simulink model "UAVtree21"  (R2019b)
settings: Solver=FixedStepAuto  StartTime=0.0  StopTime=50  RelTol=1e-3
undefined symbols (not defined in the file or in its folder): DiscIntNeverNeededParam
libraries: simulink x5, vrlib x4, robotcorelib x1
settings Model: Creator=Tesla  LastModifiedBy=Tesla
settings OptimizationCC: OptimizeBlockIOStorage=off  BufferReuse=off  GlobalBufferReuse=off  ExpressionFolding=off  LocalBlockOutputs=off  OptimizeDataStoreBuffers=off  BusAssignmentInplaceUpdate=off
settings DebuggingCC: SFUnexpectedBacktrackingDiag=warning  SFNoUnconditionalDefaultTransitionDiag=warning  UnderSpecifiedDimensionMsg=warning
settings RTWCC: GenerateReport=on  BuildConfiguration=Debug  LaunchReport=on  TargetLang=C++
settings CodeAppCC: ForceParamTrailComments=on  MATLABSourceComments=on  EnableCustomComments=on
settings GRTTargetCC: TargetLangStandard=C++03 (ISO)  CombineSignalStateStructs=on  MultiInstanceERTCode=on  CodeInterfacePackaging=C++ class  SupportVariableSizeSignals=on  MultiInstanceErrorCode=Warning

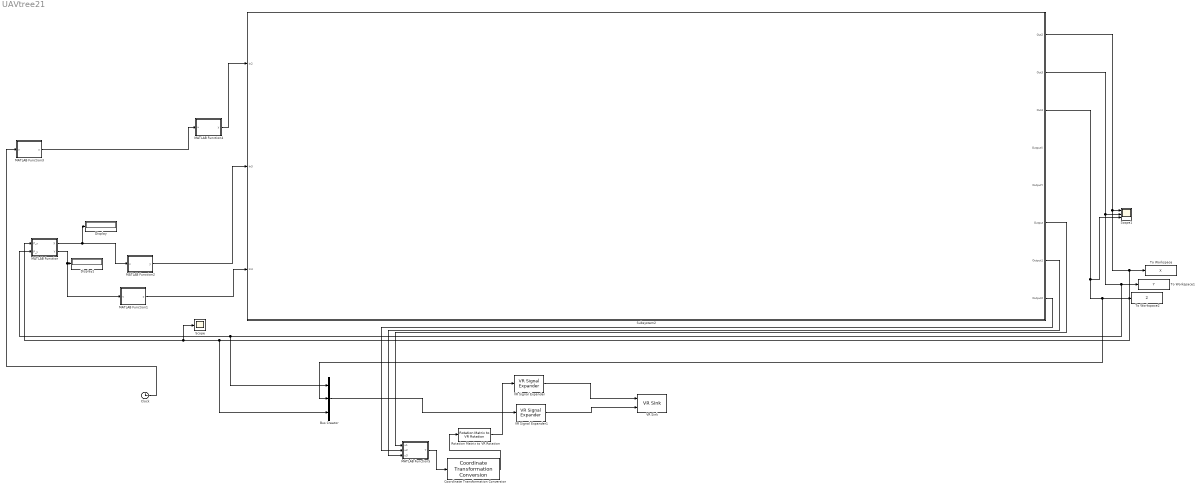
== system UAVtree21 ==
  Bus Creator : BusCreator  Inputs=3
  Clock : Clock
  Coordinate Transformation Conversion : robotcorelib/Coordinate Transformation Conversion  InputRepresentation=Euler Angles  InputEulerSequence=XYZ  ShowTrVecInputPort=on  OutputRepresentation=Rotation Matrix  OutputEulerSequence=ZYX  ShowTrVecOutputPort=on  SimulateUsing=Interpreted execution
      settings: SourceProductBaseCode=RO
  Display : Display
  Display1 : Display
  MATLAB Function : MATLAB Function  TreatAsAtomicUnit=on
  MATLAB Function1 : MATLAB Function  TreatAsAtomicUnit=on
  MATLAB Function2 : MATLAB Function  TreatAsAtomicUnit=on
  MATLAB Function3 : MATLAB Function  TreatAsAtomicUnit=on
  MATLAB Function4 : MATLAB Function  TreatAsAtomicUnit=on
  MATLAB Function5 : MATLAB Function  TreatAsAtomicUnit=on
  Rotation Matrix to VR Rotation : vrlib/Utilities/Rotation Matrix to VR Rotation  maxzero=1e-5
      settings: SourceProductName=Simulink  SourceProductBaseCode=SL
  Scope : Scope
  Scope1 : Scope  NumInputPorts=3
  Subsystem2 : Subsystem
  To Workspace : ToWorkspace  VariableName=X  SampleTime=-1
  To Workspace1 : ToWorkspace  VariableName=Y  SampleTime=-1
  To Workspace2 : ToWorkspace  VariableName=Z  SampleTime=-1
  VR Signal Expander : vrlib/VR Signal Expander  outwidth=4  outidx=[1 2 3 4]
      settings: SourceProductName=Simulink
  VR Signal Expander1 : vrlib/VR Signal Expander  outwidth=3  outidx=[1 2 3]
      settings: SourceProductName=Simulink
  VR Sink : vrlib/VR Sink  InstantiateOnLoad=on  SampleTime=0.005  ViewEnable=on  RemoteChange=off  RemoteView=off  FieldsWritten=vehicle.rotation.4.1.1.double#vehicle.translation.3.1.1.double  WorldFileName=advance.wrl  AutoView=on  VideoDimensions=[]  AllowVariableSize=off
      settings: SourceProductName=Simulink
  wires:
  Subsystem2/2(Out3) -> Scope1/2, Bus Creator/1, MATLAB Function/2(P_y), To Workspace1/1
  Subsystem2/3(Out4) -> Bus Creator/2, To Workspace2/1, Scope1/3
  MATLAB Function/2(Y) -> MATLAB Function1/1(u), Display1/1
  MATLAB Function/1(X) -> MATLAB Function2/1(u), Display/1
  MATLAB Function1/1(y) -> Subsystem2/3(In4)
  MATLAB Function2/1(y) -> Subsystem2/2(In3)
  Subsystem2/1(Out2) -> Scope1/1, Bus Creator/3, MATLAB Function/1(P_x), Scope/1, To Workspace/1
  Clock/1 -> MATLAB Function3/1(u)
  MATLAB Function3/1(y) -> MATLAB Function4/1(u)
  MATLAB Function4/1(y) -> Subsystem2/1(In2)
  Bus Creator/1 -> VR Signal Expander1/1
  Subsystem2/6(Output) -> MATLAB Function5/1(u1)
  Subsystem2/7(Output1) -> MATLAB Function5/3(u3)
  Subsystem2/8(Output2) -> MATLAB Function5/2(u2)
  MATLAB Function5/1(Y) -> Coordinate Transformation Conversion/1
  Rotation Matrix to VR Rotation/1 -> VR Signal Expander/1
  Coordinate Transformation Conversion/1 -> Rotation Matrix to VR Rotation/1
  VR Signal Expander/1 -> VR Sink/1
  VR Signal Expander1/1 -> VR Sink/2

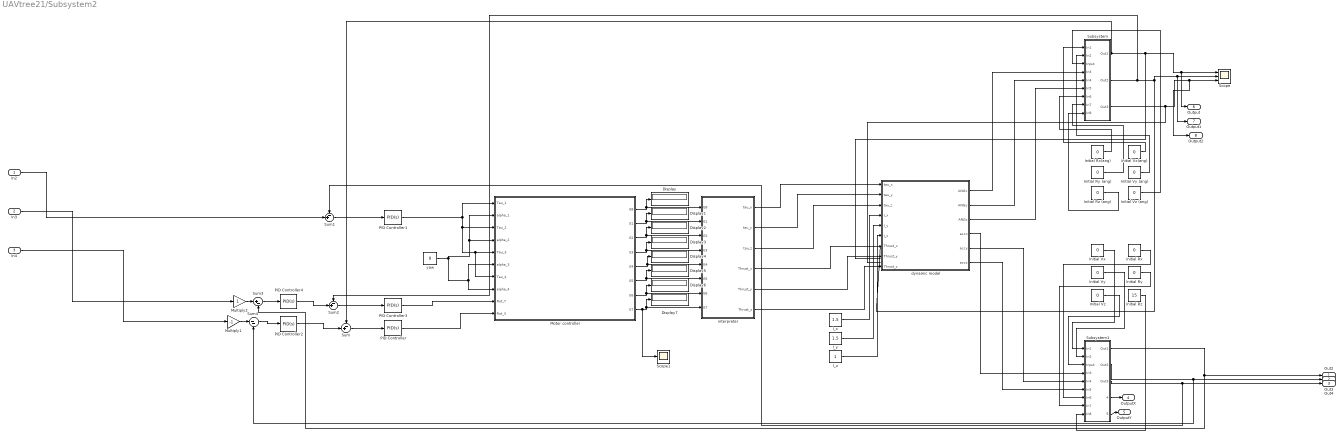
== system UAVtree21/Subsystem2 ==
  In2 : Inport
  In3 : Inport  Port=2
  In4 : Inport  Port=3
  Display{,1..7} (8 alike) : Display
  I_x : Constant  Value=1.5
  I_y : Constant  Value=1.5
  I_z : Constant
  Initial Rx : Constant  Value=0
  Initial Rx(ang) : Constant  Value=0
  Initial Ry : Constant  Value=0
  Initial Ry (ang) : Constant  Value=0
  Initial Rz : Constant  Value=15
  Initial Rz (ang) : Constant  Value=0
  Initial Vx : Constant  Value=0
  Initial Vx(ang) : Constant  Value=0
  "Initial Vy " : Constant  Value=0
  Initial Vy (ang) : Constant  Value=0
  Initial Vz : Constant  Value=0
  Initial Vz (ang) : Constant  Value=0
  Motor controller : Subsystem
  Multiply1 : Gain  Gain=-1
  Multiply2 : Gain
  PID Controller : simulink/Continuous/PID Controller  Controller=PID  Form=Parallel  TimeDomain=Continuous-time  SampleTime=-1  IntegratorMethod=Forward Euler  FilterMethod=Forward Euler  ControllerParametersSource=internal  P=-19  I=-5  D=-8  UseFilter=on  N=25  TunerSelectOption=Transfer Function Based (PID Tuner App)  InitialConditionSource=internal  InitialConditionForIntegrator=0  InitialConditionForFilter=0  DifferentiatorICPrevScaledInput=0  ExternalReset=none  TrackingMode=off  Kt=1  LimitOutput=on  UpperSaturationLimit=2  LowerSaturationLimit=-2  LinearizeAsGain=on  AntiWindupMode=clamping  Kb=1  POutMin=[]  POutMax=[]  IOutMin=[]  IOutMax=[]  DOutMin=[]  DOutMax=[]  NOutMin=[]  NOutMax=[]  SumOutMin=[]  SumOutMax=[]  SaturationOutMin=[]  SaturationOutMax=[]  PParamMin=[]  PParamMax=[]  IParamMin=[]  IParamMax=[]  DParamMin=[]  DParamMax=[]  NParamMin=[]  NParamMax=[]  KbParamMin=[]  KbParamMax=[]  KtParamMin=[]  KtParamMax=[]  KbOutMin=[]  KbOutMax=[]  KtOutMin=[]  KtOutMax=[]  IntegratorOutMin=[]  IntegratorOutMax=[]  FilterOutMin=[]  FilterOutMax=[]  SumI1OutMin=[]  SumI1OutMax=[]  SumI2OutMin=[]  SumI2OutMax=[]  SumI3OutMin=[]  SumI3OutMax=[]  SumI4OutMin=[]  SumI4OutMax=[]  SumDOutMin=[]  SumDOutMax=[]  DifferentiatorOutMin=[]  DifferentiatorOutMax=[]  FilterDiffOutCoefMin=[]  FilterDiffOutCoefMax=[]  ReciprocalOutMin=[]  ReciprocalOutMax=[]  SumDenOutMin=[]  SumDenOutMax=[]  SumNumOutMin=[]  SumNumOutMax=[]  DivideOutMin=[]  DivideOutMax=[]  IntegratorContinuousStateAttributes=''  IntegratorStateMustResolveToSignalObject=off  IntegratorRTWStateStorageClass=Auto  FilterContinuousStateAttributes=''  FilterStateMustResolveToSignalObject=off  FilterRTWStateStorageClass=Auto  ParallelPVariant=InternalParameters  IdealPVariant=Disabled  IVariant=InternalParameters  DVariant=InternalParameters  IntegratorVariant=Continuous  SatVariant=Enabled  AWVariant=ContClampingParallel  PCopyVariant=Disabled  TRVariant=Disabled  FdbkBlocksVariant=Forward  IdealPFdbkVariant=Disabled  SatFdbkVariant=Disabled  DerivativeFilterVariant=ContFilter  NVariant=InternalParameters  NCopyVariant=Disabled  FilterICVariant=InternalICsFilter  IntegratorICVariant=InternalICs  ExternalResetVariant=Disabled  TRSumVariant=Passthrough  SumFdbkVariant=Disabled  SumVariant=Sum_PID
  PID Controller1 : simulink/Continuous/PID Controller  Controller=PID  Form=Parallel  TimeDomain=Continuous-time  SampleTime=-1  IntegratorMethod=Forward Euler  FilterMethod=Forward Euler  ControllerParametersSource=internal  P=65  I=50  D=40  UseFilter=on  N=25  TunerSelectOption=Frequency Response Based  InitialConditionSource=internal  InitialConditionForIntegrator=0  InitialConditionForFilter=0  DifferentiatorICPrevScaledInput=0  ExternalReset=none  TrackingMode=off  Kt=1  LimitOutput=on  UpperSaturationLimit=12  LowerSaturationLimit=0  LinearizeAsGain=off  AntiWindupMode=clamping  Kb=1  POutMin=[]  POutMax=[]  IOutMin=[]  IOutMax=[]  DOutMin=[]  DOutMax=[]  NOutMin=[]  NOutMax=[]  SumOutMin=[]  SumOutMax=[]  SaturationOutMin=[]  SaturationOutMax=[]  PParamMin=[]  PParamMax=[]  IParamMin=[]  IParamMax=[]  DParamMin=[]  DParamMax=[]  NParamMin=[]  NParamMax=[]  KbParamMin=[]  KbParamMax=[]  KtParamMin=[]  KtParamMax=[]  KbOutMin=[]  KbOutMax=[]  KtOutMin=[]  KtOutMax=[]  IntegratorOutMin=[]  IntegratorOutMax=[]  FilterOutMin=[]  FilterOutMax=[]  SumI1OutMin=[]  SumI1OutMax=[]  SumI2OutMin=[]  SumI2OutMax=[]  SumI3OutMin=[]  SumI3OutMax=[]  SumI4OutMin=[]  SumI4OutMax=[]  SumDOutMin=[]  SumDOutMax=[]  DifferentiatorOutMin=[]  DifferentiatorOutMax=[]  FilterDiffOutCoefMin=[]  FilterDiffOutCoefMax=[]  ReciprocalOutMin=[]  ReciprocalOutMax=[]  SumDenOutMin=[]  SumDenOutMax=[]  SumNumOutMin=[]  SumNumOutMax=[]  DivideOutMin=[]  DivideOutMax=[]  IntegratorContinuousStateAttributes=''  IntegratorStateMustResolveToSignalObject=off  IntegratorRTWStateStorageClass=Auto  FilterContinuousStateAttributes=''  FilterStateMustResolveToSignalObject=off  FilterRTWStateStorageClass=Auto  ParallelPVariant=InternalParameters  IdealPVariant=Disabled  IVariant=InternalParameters  DVariant=InternalParameters  IntegratorVariant=Continuous  SatVariant=Enabled  AWVariant=ContClampingParallel  PCopyVariant=Disabled  TRVariant=Disabled  FdbkBlocksVariant=Forward  IdealPFdbkVariant=Disabled  SatFdbkVariant=Disabled  DerivativeFilterVariant=ContFilter  NVariant=InternalParameters  NCopyVariant=Disabled  FilterICVariant=InternalICsFilter  IntegratorICVariant=InternalICs  ExternalResetVariant=Disabled  TRSumVariant=Passthrough  SumFdbkVariant=Disabled  SumVariant=Sum_PID
  PID Controller2 : simulink/Continuous/PID Controller  Controller=PID  Form=Parallel  TimeDomain=Continuous-time  SampleTime=-1  IntegratorMethod=Forward Euler  FilterMethod=Forward Euler  ControllerParametersSource=internal  P=-0.3  I=-0.01  D=-0.025  UseFilter=on  N=100  TunerSelectOption=Transfer Function Based (PID Tuner App)  InitialConditionSource=internal  InitialConditionForIntegrator=0  InitialConditionForFilter=0  DifferentiatorICPrevScaledInput=0  ExternalReset=none  TrackingMode=off  Kt=1  LimitOutput=on  UpperSaturationLimit=1  LowerSaturationLimit=-1  LinearizeAsGain=on  AntiWindupMode=clamping  Kb=1  POutMin=[]  POutMax=[]  IOutMin=[]  IOutMax=[]  DOutMin=[]  DOutMax=[]  NOutMin=[]  NOutMax=[]  SumOutMin=[]  SumOutMax=[]  SaturationOutMin=[]  SaturationOutMax=[]  PParamMin=[]  PParamMax=[]  IParamMin=[]  IParamMax=[]  DParamMin=[]  DParamMax=[]  NParamMin=[]  NParamMax=[]  KbParamMin=[]  KbParamMax=[]  KtParamMin=[]  KtParamMax=[]  KbOutMin=[]  KbOutMax=[]  KtOutMin=[]  KtOutMax=[]  IntegratorOutMin=[]  IntegratorOutMax=[]  FilterOutMin=[]  FilterOutMax=[]  SumI1OutMin=[]  SumI1OutMax=[]  SumI2OutMin=[]  SumI2OutMax=[]  SumI3OutMin=[]  SumI3OutMax=[]  SumI4OutMin=[]  SumI4OutMax=[]  SumDOutMin=[]  SumDOutMax=[]  DifferentiatorOutMin=[]  DifferentiatorOutMax=[]  FilterDiffOutCoefMin=[]  FilterDiffOutCoefMax=[]  ReciprocalOutMin=[]  ReciprocalOutMax=[]  SumDenOutMin=[]  SumDenOutMax=[]  SumNumOutMin=[]  SumNumOutMax=[]  DivideOutMin=[]  DivideOutMax=[]  IntegratorContinuousStateAttributes=''  IntegratorStateMustResolveToSignalObject=off  IntegratorRTWStateStorageClass=Auto  FilterContinuousStateAttributes=''  FilterStateMustResolveToSignalObject=off  FilterRTWStateStorageClass=Auto  ParallelPVariant=InternalParameters  IdealPVariant=Disabled  IVariant=InternalParameters  DVariant=InternalParameters  IntegratorVariant=Continuous  SatVariant=Enabled  AWVariant=ContClampingParallel  PCopyVariant=Disabled  TRVariant=Disabled  FdbkBlocksVariant=Forward  IdealPFdbkVariant=Disabled  SatFdbkVariant=Disabled  DerivativeFilterVariant=ContFilter  NVariant=InternalParameters  NCopyVariant=Disabled  FilterICVariant=InternalICsFilter  IntegratorICVariant=InternalICs  ExternalResetVariant=Disabled  TRSumVariant=Passthrough  SumFdbkVariant=Disabled  SumVariant=Sum_PID
  PID Controller3 : simulink/Continuous/PID Controller  Controller=PID  Form=Parallel  TimeDomain=Continuous-time  SampleTime=-1  IntegratorMethod=Forward Euler  FilterMethod=Forward Euler  ControllerParametersSource=internal  P=19  I=5  D=8  UseFilter=on  N=25  TunerSelectOption=Transfer Function Based (PID Tuner App)  InitialConditionSource=internal  InitialConditionForIntegrator=0  InitialConditionForFilter=0  DifferentiatorICPrevScaledInput=0  ExternalReset=none  TrackingMode=off  Kt=1  LimitOutput=on  UpperSaturationLimit=2  LowerSaturationLimit=-2  LinearizeAsGain=on  AntiWindupMode=clamping  Kb=1  POutMin=[]  POutMax=[]  IOutMin=[]  IOutMax=[]  DOutMin=[]  DOutMax=[]  NOutMin=[]  NOutMax=[]  SumOutMin=[]  SumOutMax=[]  SaturationOutMin=[]  SaturationOutMax=[]  PParamMin=[]  PParamMax=[]  IParamMin=[]  IParamMax=[]  DParamMin=[]  DParamMax=[]  NParamMin=[]  NParamMax=[]  KbParamMin=[]  KbParamMax=[]  KtParamMin=[]  KtParamMax=[]  KbOutMin=[]  KbOutMax=[]  KtOutMin=[]  KtOutMax=[]  IntegratorOutMin=[]  IntegratorOutMax=[]  FilterOutMin=[]  FilterOutMax=[]  SumI1OutMin=[]  SumI1OutMax=[]  SumI2OutMin=[]  SumI2OutMax=[]  SumI3OutMin=[]  SumI3OutMax=[]  SumI4OutMin=[]  SumI4OutMax=[]  SumDOutMin=[]  SumDOutMax=[]  DifferentiatorOutMin=[]  DifferentiatorOutMax=[]  FilterDiffOutCoefMin=[]  FilterDiffOutCoefMax=[]  ReciprocalOutMin=[]  ReciprocalOutMax=[]  SumDenOutMin=[]  SumDenOutMax=[]  SumNumOutMin=[]  SumNumOutMax=[]  DivideOutMin=[]  DivideOutMax=[]  IntegratorContinuousStateAttributes=''  IntegratorStateMustResolveToSignalObject=off  IntegratorRTWStateStorageClass=Auto  FilterContinuousStateAttributes=''  FilterStateMustResolveToSignalObject=off  FilterRTWStateStorageClass=Auto  ParallelPVariant=InternalParameters  IdealPVariant=Disabled  IVariant=InternalParameters  DVariant=InternalParameters  IntegratorVariant=Continuous  SatVariant=Enabled  AWVariant=ContClampingParallel  PCopyVariant=Disabled  TRVariant=Disabled  FdbkBlocksVariant=Forward  IdealPFdbkVariant=Disabled  SatFdbkVariant=Disabled  DerivativeFilterVariant=ContFilter  NVariant=InternalParameters  NCopyVariant=Disabled  FilterICVariant=InternalICsFilter  IntegratorICVariant=InternalICs  ExternalResetVariant=Disabled  TRSumVariant=Passthrough  SumFdbkVariant=Disabled  SumVariant=Sum_PID
  PID Controller4 : simulink/Continuous/PID Controller  Controller=PID  Form=Parallel  TimeDomain=Continuous-time  SampleTime=-1  IntegratorMethod=Forward Euler  FilterMethod=Forward Euler  ControllerParametersSource=internal  P=-0.3  I=-0.01  D=-0.025  UseFilter=on  N=150  TunerSelectOption=Transfer Function Based (PID Tuner App)  InitialConditionSource=internal  InitialConditionForIntegrator=0  InitialConditionForFilter=0  DifferentiatorICPrevScaledInput=0  ExternalReset=none  TrackingMode=off  Kt=1  LimitOutput=on  UpperSaturationLimit=1  LowerSaturationLimit=-1  LinearizeAsGain=off  AntiWindupMode=clamping  Kb=1  POutMin=[]  POutMax=[]  IOutMin=[]  IOutMax=[]  DOutMin=[]  DOutMax=[]  NOutMin=[]  NOutMax=[]  SumOutMin=[]  SumOutMax=[]  SaturationOutMin=[]  SaturationOutMax=[]  PParamMin=[]  PParamMax=[]  IParamMin=[]  IParamMax=[]  DParamMin=[]  DParamMax=[]  NParamMin=[]  NParamMax=[]  KbParamMin=[]  KbParamMax=[]  KtParamMin=[]  KtParamMax=[]  KbOutMin=[]  KbOutMax=[]  KtOutMin=[]  KtOutMax=[]  IntegratorOutMin=[]  IntegratorOutMax=[]  FilterOutMin=[]  FilterOutMax=[]  SumI1OutMin=[]  SumI1OutMax=[]  SumI2OutMin=[]  SumI2OutMax=[]  SumI3OutMin=[]  SumI3OutMax=[]  SumI4OutMin=[]  SumI4OutMax=[]  SumDOutMin=[]  SumDOutMax=[]  DifferentiatorOutMin=[]  DifferentiatorOutMax=[]  FilterDiffOutCoefMin=[]  FilterDiffOutCoefMax=[]  ReciprocalOutMin=[]  ReciprocalOutMax=[]  SumDenOutMin=[]  SumDenOutMax=[]  SumNumOutMin=[]  SumNumOutMax=[]  DivideOutMin=[]  DivideOutMax=[]  IntegratorContinuousStateAttributes=''  IntegratorStateMustResolveToSignalObject=off  IntegratorRTWStateStorageClass=Auto  FilterContinuousStateAttributes=''  FilterStateMustResolveToSignalObject=off  FilterRTWStateStorageClass=Auto  ParallelPVariant=InternalParameters  IdealPVariant=Disabled  IVariant=InternalParameters  DVariant=InternalParameters  IntegratorVariant=Continuous  SatVariant=Enabled  AWVariant=ContClampingParallel  PCopyVariant=Disabled  TRVariant=Disabled  FdbkBlocksVariant=Forward  IdealPFdbkVariant=Disabled  SatFdbkVariant=Disabled  DerivativeFilterVariant=ContFilter  NVariant=InternalParameters  NCopyVariant=Disabled  FilterICVariant=InternalICsFilter  IntegratorICVariant=InternalICs  ExternalResetVariant=Disabled  TRSumVariant=Passthrough  SumFdbkVariant=Disabled  SumVariant=Sum_PID
  Scope : Scope  NumInputPorts=3
  Scope1 : Scope
  Subsystem : Subsystem
  Subsystem1 : Subsystem
  Sum : Sum  Inputs=-+|
  Sum1 : Sum  Inputs=-+|
  Sum2 : Sum  Inputs=-+|
  Sum3 : Sum  Inputs=|+-
  Sum4 : Sum  Inputs=|--
  dynamic model : MATLAB Function  TreatAsAtomicUnit=on
  interpreter : MATLAB Function  TreatAsAtomicUnit=on
  yaw : Constant  Value=0
  Out2 : Outport
  Out3 : Outport  Port=2
  Out4 : Outport  Port=3
  OutputX : Outport  Port=4
  OutputY : Outport  Port=5
  Output : Outport  Port=6
  Output1 : Outport  Port=7
  Output2 : Outport  Port=8
  wires:
  In3/1 -> Multiply2/1
  "Initial Vy "/1 -> Subsystem1/2(In2)
  Motor controller/2(E1) -> Display1/1, interpreter/2(E1)
  PID Controller1/1 -> Motor controller/5(Tau_3), Motor controller/7(Tau_4), Motor controller/3(Tau_2), Motor controller/1("Tau_1 ")
  Initial Rx(ang)/1 -> Subsystem/7(In6)
  Sum/1 -> PID Controller/1
  Subsystem1/2(Out2) -> Out3/1, Sum4/2
  Motor controller/5(E4) -> Display4/1, interpreter/5(E4)
  Subsystem1/1(Out1) -> Out2/1, Sum3/2
  Initial Vz/1 -> Subsystem1/3(Input)
  PID Controller2/1 -> Sum/2
  PID Controller/1 -> Motor controller/10(Rot_X)
  Motor controller/6(E5) -> Display5/1, interpreter/6(E5)
  Initial Vx(ang)/1 -> Subsystem/1(In1)
  dynamic model/2(ANGy) -> Subsystem/5(In4)
  dynamic model/4(accx) -> Subsystem1/4(In3)
  Subsystem/2(Out2) -> Sum2/1, Scope/2, Output1/1
  dynamic model/6(accz) -> Subsystem1/6(In5)
  Subsystem1/3(Out3) -> Out4/1, Sum1/1
  I_z/1 -> dynamic model/6(I_z)
  PID Controller4/1 -> Sum2/2
  Sum3/1 -> PID Controller4/1
  Initial Ry/1 -> Subsystem1/8(In7)
  Initial Vz (ang)/1 -> Subsystem/3(Input)
  Motor controller/1("E8 ") -> Display/1, interpreter/1(E8)
  Sum1/1 -> PID Controller1/1
  interpreter/1(tau_x) -> dynamic model/1(tau_x)
  Initial Vx/1 -> Subsystem1/1(In1)
  In4/1 -> Multiply1/1
  Initial Ry (ang)/1 -> Subsystem/8(In7)
  Subsystem/1(Out1) -> Scope/1, Output/1, Sum/1
  I_y/1 -> dynamic model/5(I_y)
  Sum2/1 -> PID Controller3/1
  Motor controller/7(E6) -> Display6/1, interpreter/7(E6)
  dynamic model/3(ANGz) -> Subsystem/6(In5)
  Sum4/1 -> PID Controller2/1
  Motor controller/8(E7) -> Scope1/1, Display7/1, interpreter/8(E7)
  Initial Rx/1 -> Subsystem1/7(In6)
  I_x/1 -> dynamic model/4(I_x)
  dynamic model/5(accy) -> Subsystem1/5(In4)
  PID Controller3/1 -> Motor controller/9(Rot_Y)
  Multiply1/1 -> Sum4/1
  interpreter/5(Thrust_y) -> dynamic model/8(Thrust_y)
  interpreter/2(tau_y) -> dynamic model/2(tau_y)
  interpreter/4(Thrust_x) -> dynamic model/7(Thrust_x)
  Motor controller/3(E2) -> Display2/1, interpreter/3(E2)
  Initial Rz (ang)/1 -> Subsystem/9(In8)
  yaw/1 -> Motor controller/8(alpha_4), Motor controller/6(alpha_3), Motor controller/4(alpha_2), Motor controller/2(alpha_1)
  interpreter/3(tau_z) -> dynamic model/3(tau_z)
  Initial Rz/1 -> Subsystem1/9(In8)
  interpreter/6(Thrust_z) -> dynamic model/9(Thrust_z)
  Initial Vy (ang)/1 -> Subsystem/2(In2)
  Motor controller/4(E3) -> Display3/1, interpreter/4(E3)
  Multiply2/1 -> Sum3/1
  dynamic model/1(ANGx) -> Subsystem/4(In3)
  In2/1 -> Sum1/2
  Subsystem1/4(Output) -> OutputX/1
  Subsystem1/5(Output1) -> OutputY/1
  Subsystem/3(Out3) -> Output2/1, Scope/3

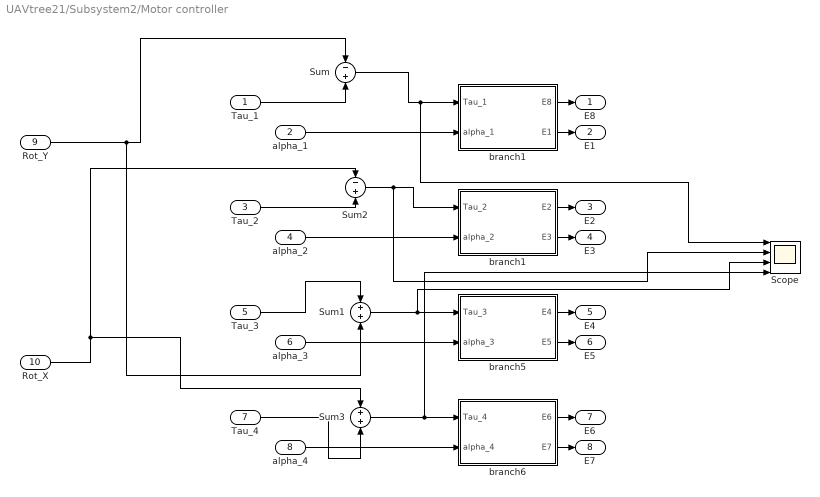
== system UAVtree21/Subsystem2/Motor controller ==
  "Tau_1 " : Inport
  alpha_1 : Inport  Port=2
  Tau_2 : Inport  Port=3
  alpha_2 : Inport  Port=4
  Tau_3 : Inport  Port=5
  alpha_3 : Inport  Port=6
  Tau_4 : Inport  Port=7
  alpha_4 : Inport  Port=8
  Rot_Y : Inport  Port=9
  Rot_X : Inport  Port=10
  Scope : Scope  NumInputPorts=4
  Sum : Sum  Inputs=-|+
  Sum1 : Sum  Inputs=+|+
  Sum2 : Sum  Inputs=-|+
  Sum3 : Sum  Inputs=+|+
  branch1 : MATLAB Function  TreatAsAtomicUnit=on
  "branch1 " : MATLAB Function  TreatAsAtomicUnit=on
  branch5 : MATLAB Function  TreatAsAtomicUnit=on
  branch6 : MATLAB Function  TreatAsAtomicUnit=on
  "E8 " : Outport
  E1 : Outport  Port=2
  E2 : Outport  Port=3
  E3 : Outport  Port=4
  E4 : Outport  Port=5
  E5 : Outport  Port=6
  E6 : Outport  Port=7
  E7 : Outport  Port=8
  wires:
  Sum/1 -> Scope/1, "branch1 "/1(Tau_1)
  Sum3/1 -> Scope/4, branch6/1(Tau_4)
  Rot_X/1 -> Sum2/1, Sum3/1
  Tau_4/1 -> Sum3/2
  Tau_2/1 -> Sum2/2
  Tau_3/1 -> Sum1/1
  Sum2/1 -> Scope/2, branch1/1(Tau_2)
  alpha_2/1 -> branch1/2(alpha_2)
  branch6/1(E6) -> E6/1
  Rot_Y/1 -> Sum1/2, Sum/1
  Sum1/1 -> Scope/3, branch5/1(Tau_3)
  "Tau_1 "/1 -> Sum/2
  alpha_4/1 -> branch6/2(alpha_4)
  alpha_1/1 -> "branch1 "/2(alpha_1)
  alpha_3/1 -> branch5/2(alpha_3)
  branch1/2(E3) -> E3/1
  branch1/1(E2) -> E2/1
  "branch1 "/1(E8) -> "E8 "/1
  "branch1 "/2(E1) -> E1/1
  branch5/2(E5) -> E5/1
  branch6/2(E7) -> E7/1
  branch5/1(E4) -> E4/1

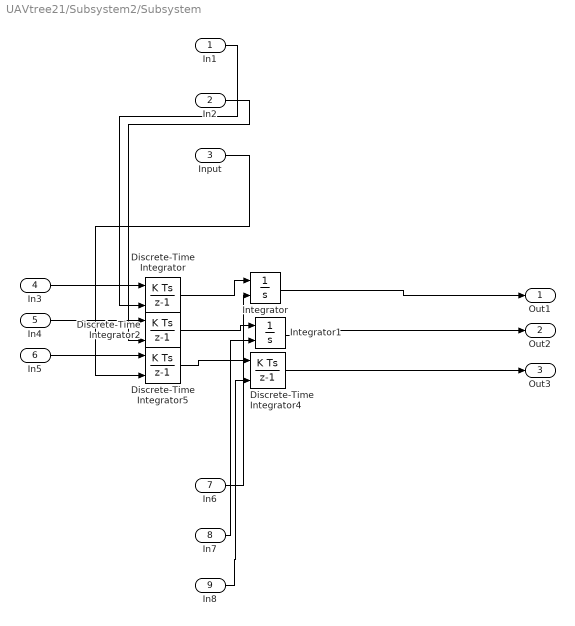
== system UAVtree21/Subsystem2/Subsystem ==
  In1 : Inport
  In2 : Inport  Port=2
  Input : Inport  Port=3
  In3 : Inport  Port=4
  In4 : Inport  Port=5
  In5 : Inport  Port=6
  In6 : Inport  Port=7
  In7 : Inport  Port=8
  In8 : Inport  Port=9
  Discrete-Time Integrator : DiscreteIntegrator  InitialConditionSource=external  SampleTime=0.01  ICPrevOutput=DiscIntNeverNeededParam  ICPrevScaledInput=DiscIntNeverNeededParam
  Discrete-Time Integrator2 : DiscreteIntegrator  InitialConditionSource=external  SampleTime=-1  ICPrevOutput=DiscIntNeverNeededParam  ICPrevScaledInput=DiscIntNeverNeededParam
  Discrete-Time Integrator4 : DiscreteIntegrator  InitialConditionSource=external  SampleTime=-1  ICPrevOutput=DiscIntNeverNeededParam  ICPrevScaledInput=DiscIntNeverNeededParam
  Discrete-Time Integrator5 : DiscreteIntegrator  InitialConditionSource=external  SampleTime=-1  ICPrevOutput=DiscIntNeverNeededParam  ICPrevScaledInput=DiscIntNeverNeededParam
  Integrator : Integrator  InitialConditionSource=external
  Integrator1 : Integrator  InitialConditionSource=external
  Out1 : Outport
  Out2 : Outport  Port=2
  Out3 : Outport  Port=3
  wires:
  In5/1 -> Discrete-Time Integrator5/1
  Discrete-Time Integrator4/1 -> Out3/1
  Discrete-Time Integrator2/1 -> Integrator1/1
  In6/1 -> Integrator/2
  Input/1 -> Discrete-Time Integrator5/2
  Discrete-Time Integrator5/1 -> Discrete-Time Integrator4/1
  In8/1 -> Discrete-Time Integrator4/2
  Discrete-Time Integrator/1 -> Integrator/1
  Integrator/1 -> Out1/1
  Integrator1/1 -> Out2/1
  In4/1 -> Discrete-Time Integrator2/1
  In7/1 -> Integrator1/2
  In2/1 -> Discrete-Time Integrator2/2
  In3/1 -> Discrete-Time Integrator/1
  In1/1 -> Discrete-Time Integrator/2

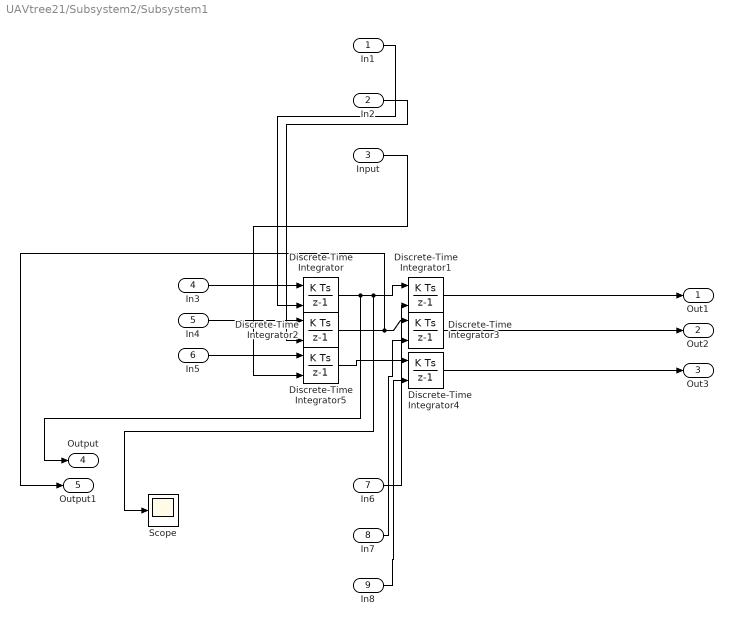
== system UAVtree21/Subsystem2/Subsystem1 ==
  In1 : Inport
  In2 : Inport  Port=2
  Input : Inport  Port=3
  In3 : Inport  Port=4
  In4 : Inport  Port=5
  In5 : Inport  Port=6
  In6 : Inport  Port=7
  In7 : Inport  Port=8
  In8 : Inport  Port=9
  Discrete-Time Integrator : DiscreteIntegrator  InitialConditionSource=external  SampleTime=0.01  ICPrevOutput=DiscIntNeverNeededParam  ICPrevScaledInput=DiscIntNeverNeededParam
  Discrete-Time Integrator{1..5} (5 alike) : DiscreteIntegrator  InitialConditionSource=external  SampleTime=-1  ICPrevOutput=DiscIntNeverNeededParam  ICPrevScaledInput=DiscIntNeverNeededParam
  Scope : Scope
  Out1 : Outport
  Out2 : Outport  Port=2
  Out3 : Outport  Port=3
  Output : Outport  Port=4
  Output1 : Outport  Port=5
  wires:
  In5/1 -> Discrete-Time Integrator5/1
  Discrete-Time Integrator4/1 -> Out3/1
  Discrete-Time Integrator2/1 -> Output1/1, Discrete-Time Integrator3/1
  In6/1 -> Discrete-Time Integrator1/2
  Input/1 -> Discrete-Time Integrator5/2
  Discrete-Time Integrator5/1 -> Discrete-Time Integrator4/1
  In8/1 -> Discrete-Time Integrator4/2
  Discrete-Time Integrator/1 -> Output/1, Scope/1, Discrete-Time Integrator1/1
  Discrete-Time Integrator1/1 -> Out1/1
  Discrete-Time Integrator3/1 -> Out2/1
  In4/1 -> Discrete-Time Integrator2/1
  In7/1 -> Discrete-Time Integrator3/2
  In2/1 -> Discrete-Time Integrator2/2
  In3/1 -> Discrete-Time Integrator/1
  In1/1 -> Discrete-Time Integrator/2

== matlab function UAVtree21/Subsystem2/dynamic model ==
  data: tau_x input; ANGx output; tau_y input; tau_z input; I_x input; I_y input; I_z input; Thrust_x input; Thrust_y input; Thrust_z input; ANGy output; ANGz output; accx output; accy output; accz output
function [ANGx, ANGy, ANGz, accx ,accy, accz] = fcn(tau_x, tau_y, tau_z, I_x, I_y, I_z,Thrust_x,Thrust_y,Thrust_z)

mass = 1;
g = -5;
ANG = [tau_x/I_x;tau_y/I_y;tau_z/I_z];

ANGx = ANG(1);
ANGy = ANG(2);
ANGz = ANG(3);

acc = [(Thrust_x/mass);(Thrust_y/mass);(Thrust_z/mass)];
accx = acc(1);
accy = acc(2);
accz = acc(3);
end

== matlab function UAVtree21/Subsystem2/Motor controller/branch1  ==
  data: Tau_1 input; E8 output; alpha_1 input; E1 output
function[E8, E1] = fcn(Tau_1, alpha_1)
    E8 = (Tau_1 - (alpha_1*Tau_1))*0.5;
    E1 = (Tau_1 + (alpha_1*Tau_1))*0.5;
end

== matlab function UAVtree21/Subsystem2/interpreter ==
  data: E8 input; tau_x output; E1 input; E2 input; E3 input; E4 input; E5 input; E6 input; E7 input; tau_y output; tau_z output; Thrust_x output; Thrust_y output; Thrust_z output
function [tau_x, tau_y, tau_z, Thrust_x, Thrust_y, Thrust_z] = fcn(E8, E1, E2, E3, E4, E5, E6, E7)

tau_x = ((E2+E3)-(E6+E7)) + 0.1*((E1+E4)-(E5+E8));
tau_y = ((E4+E5)-(E1+E8)) + 0.1*((E3+E6)-(E2+E7));
tau_z = (0.1*(E2+E6+E8+E4) - 0.1*(E3+E7+E1+E5));

Thrust_z = E1+E2+E3+E4+E5+E6+E7+E8;
Thrust_y = (0.1*(E5+E8)) - (0.1*(E4+E1));
Thrust_x = (0.1*(E3+E6)) - (0.1*(E2+E7));

end

== matlab function UAVtree21/MATLAB Function ==
  data: X output; Y output; P_x input; P_y input
function [X,Y] = fcn(P_x, P_y)
    
    persistent y 
        if isempty(y)
        y = 1;
    end
 
   

A = [0.5 -1; 6 5]
X = A(y,1)
Y = A(y,2)
E_x = X - P_x;
E_y = Y - P_y;
E = abs(E_x + E_y);

            if (E > 0.07)
                y = y;
       
            else if ((y+1) > 2) 
                y = y;
                
                
            else        
                y = y+1;
                
            end  
        
            
end

== matlab function UAVtree21/Subsystem2/Motor controller/branch1 ==
  data: Tau_2 input; E2 output; alpha_2 input; E3 output
function[E2, E3] = fcn(Tau_2, alpha_2)
    E2 = (Tau_2 - (alpha_2*Tau_2))*0.5;
    E3 = (Tau_2 + (alpha_2*Tau_2))*0.5;
end

== matlab function UAVtree21/Subsystem2/Motor controller/branch5 ==
  data: Tau_3 input; E4 output; alpha_3 input; E5 output
function[E4, E5] = fcn(Tau_3, alpha_3)
    E4 = (Tau_3 - (alpha_3*Tau_3))*0.5;
    E5 = (Tau_3 + (alpha_3*Tau_3))*0.5;
end

== matlab function UAVtree21/Subsystem2/Motor controller/branch6 ==
  data: Tau_4 input; E6 output; alpha_4 input; E7 output
function[E6, E7] = fcn(Tau_4, alpha_4)
    E6 = (Tau_4 - (alpha_4*Tau_4))*0.5;
    E7 = (Tau_4 + (alpha_4*Tau_4))*0.5;
end

== matlab function UAVtree21/MATLAB Function1 ==
  data: u input; y output
function y = fcn(u)

    persistent u_old
        if isempty(u_old)
               u_old = 0;
        end
        
        E = u - u_old;
        
        y = u_old + 0.001*E;
        u_old = y;
        

end

== matlab function UAVtree21/MATLAB Function2 ==
  data: u input; y output
function y = fcn(u)

    persistent u_old
        if isempty(u_old)
               u_old = 0;
        end
        
        E = u - u_old;
        
        y = u_old + 0.001*E;
        u_old = y;
        

end

== matlab function UAVtree21/MATLAB Function3 ==
  data: u input; y output
function y = fcn(u)

if (u > 25)
    y = 0.25
else 
    y = 5
end
end

== matlab function UAVtree21/MATLAB Function4 ==
  settings: updateMethod=DISCRETE
  data: u input; y output
function y = fcn(u)

    persistent u_old
        if isempty(u_old)
               u_old = 0;
        end
        
        E = u - u_old;
        
        y = u_old + 0.003*E;
        u_old = y;
        

end

== matlab function UAVtree21/MATLAB Function5 ==
  settings: updateMethod=DISCRETE
  data: u1 input; Y output; u2 input; u3 input
function Y = fcn(u1, u2, u3)


persistent A

    if isempty(A)
    A = [0; 0; 0];
    
    else
    A(1,1) = u1;
    A(2,1) = u2;
    A(3,1) = u3;
    end
    Y = A;
end
